simulink model "clarck"  (R2024a)
settings: Solver=FixedStepAuto  StartTime=0.0  StopTime=inf  RelTol=1e-3  EnableMultiTasking=on
libraries: stm32f4xxblockslib x1
settings Model: Creator=wsl  LastModifiedBy=wsl
settings SolverCC: AutoInsertRateTranBlk=on
settings OptimizationCC: EnhancedBackFolding=on  PassReuseOutputArgsAs=Individual arguments  ZeroExternalMemoryAtStartup=off  ZeroInternalMemoryAtStartup=off  MaxStackSize=64  OptimizeBlockOrder=speed  DifferentSizesBufferReuse=on  OptimizationCustomize=off  EfficientTunableParamExpr=on
settings DebuggingCC: ParameterTunabilityLossMsg=error
settings HardwareCC: ProdBitPerPointer=32  ProdBitPerSizeT=32  ProdBitPerPtrDiffT=32  ProdLargestAtomicInteger=Long  ProdLargestAtomicFloat=Double  ProdWordSize=32  ProdLongLongMode=on  ProdHWDeviceType=ARM Compatible->ARM Cortex-M
settings SFSimCC: MATLABDynamicMemAlloc=off
settings RTWCC: Description=Embedded Coder  SystemTargetFile=ert.tlc  HardwareBoard=STM32F4xx Based  TemplateMakefile=ert_default_tmf  Toolchain=GNU Tools for ARM Embedded Processors
settings CodeAppCC: ForceParamTrailComments=on  IgnoreCustomStorageClasses=off  OperatorAnnotations=on  SimulinkDataObjDesc=on  SFDataObjDesc=on  InsertBlockDesc=on
settings ERTTargetCC: TargetLangStandard=C99 (ISO)  CodeReplacementLibrary=ARM Cortex-M  ExtModeTransport=3  ExtModeStaticAlloc=on  ExtModeStaticAllocSize=2048  ExtModeMexFile=ext_xcp  ExtModeIntrfLevel=Level2 - Open

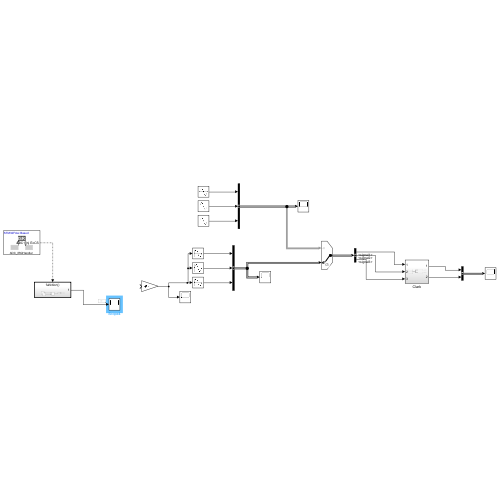
[thumbnail: Simulink's stored preview of the top-level diagram]
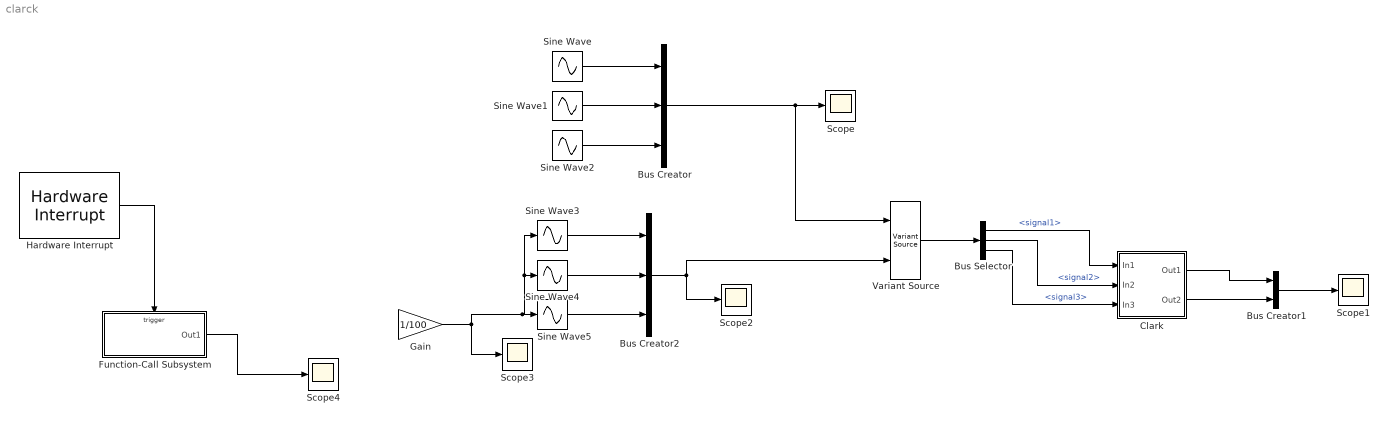
== system clarck ==
  Bus Creator : BusCreator  Inputs=3
  Bus Creator1 : BusCreator  Inputs=2
  Bus Creator2 : BusCreator  Inputs=3
  Bus Selector : BusSelector  OutputSignals=signal1,signal2,signal3
  Clark : Subsystem
  Function-Call Subsystem : Subsystem  TreatAsAtomicUnit=on
  Gain : Gain  Gain=1/100
  Hardware Interrupt : stm32f4xxblockslib/Hardware Interrupt  ISRGroup=Analog to digital converter (ADC)  ISRName=ADC_IRQHandler  ISRNumber=33  EventsList={ 'off', 'ADC1 OVR', '1'; 'off', 'ADC1 Reg EoCS', '2'; 'on', 'ADC1 Inj EoCS', '3'; 'off', 'ADC1 Watchdog', '4'; 'off', 'ADC2 OVR', '5'; 'off', 'ADC2 Reg EoCS', '6'; 'off', 'ADC2 Inj EoCS', '7'; 'off', 'ADC2 Watchdog', '8'; 'off', 'ADC3 OVR', '9'; 'off', 'ADC3 Reg EoCS', '10'; 'off', 'ADC3 Inj EoCS', '11'; 'off', 'ADC3 Watchdog', '12'; 'off', 'Custom event', '13' }  SelectedEvents={'ADC1 Inj EoCS'}  TaskPriority=30  DisablePreemption=off  ClearInterruptFlagsAtEndOfEvent=off  InterruptDefinitionFile=$(TARGET_ROOT)/registry/interrupts/STM32F4xxBased_interrupts.xml  HardwareBoard=STM32F4xx Based  EnableSimPort=off
  Scope{,1..4} (5 alike) : Scope
  Sine Wave : Sin  SineType=Sample based  Samples=1000  SampleTime=1e-4
  Sine Wave1 : Sin  SineType=Sample based  Samples=1000  SampleTime=1e-4  Offset=333
  Sine Wave2 : Sin  SineType=Sample based  Samples=1000  SampleTime=1e-4  Offset=-333
  Sine Wave3 : Sin  TimeSource=Use external signal  Frequency=2*pi  Samples=1000  SampleTime=1e-4
  Sine Wave4 : Sin  TimeSource=Use external signal  Frequency=2*pi  Phase=2/3*pi  Samples=1000  SampleTime=1e-4  Offset=333
  Sine Wave5 : Sin  TimeSource=Use external signal  Frequency=2*pi  Phase=-2/3*pi  Samples=1000  SampleTime=1e-4  Offset=-333
  Variant Source : VariantSource  VariantControlMode=sim codegen switching
  wires:
  Sine Wave/1 -> Bus Creator/1
  Bus Creator/1 -> Variant Source/1, Scope/1
  Sine Wave1/1 -> Bus Creator/2
  Sine Wave2/1 -> Bus Creator/3
  Variant Source/1 -> Bus Selector/1
  Bus Selector/1 -> Clark/1(In1)  "<signal1>"
  Bus Selector/2 -> Clark/2(In2)  "<signal2>"
  Bus Selector/3 -> Clark/3(In3)  "<signal3>"
  Clark/1(Out1) -> Bus Creator1/1
  Clark/2(Out2) -> Bus Creator1/2
  Bus Creator1/1 -> Scope1/1
  Sine Wave3/1 -> Bus Creator2/1
  Sine Wave5/1 -> Bus Creator2/3
  Sine Wave4/1 -> Bus Creator2/2
  Bus Creator2/1 -> Variant Source/2, Scope2/1
  Function-Call Subsystem/1(Out1) -> Scope4/1
  Gain/1 -> Sine Wave4/1, Sine Wave3/1, Sine Wave5/1, Scope3/1
  Hardware Interrupt/1 -> Function-Call Subsystem/Trigger

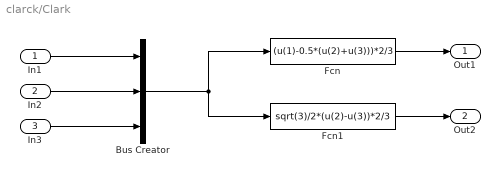
== system clarck/Clark ==
  In1 : Inport
  In2 : Inport  Port=2
  In3 : Inport  Port=3
  Bus Creator : BusCreator  Inputs=3
  Fcn : Fcn  Expr=(u(1)-0.5*(u(2)+u(3)))*2/3
  Fcn1 : Fcn  Expr=sqrt(3)/2*(u(2)-u(3))*2/3
  Out1 : Outport
  Out2 : Outport  Port=2
  wires:
  In1/1 -> Bus Creator/1
  In3/1 -> Bus Creator/3
  Fcn1/1 -> Out2/1
  In2/1 -> Bus Creator/2
  Bus Creator/1 -> Fcn1/1, Fcn/1
  Fcn/1 -> Out1/1

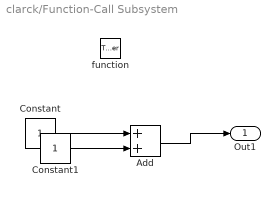
== system clarck/Function-Call Subsystem ==
  function : TriggerPort  TriggerType=function-call  VariantControl=(inherit)
  Add : Sum
  Constant : Constant
  Constant1 : Constant
  Out1 : Outport
  wires:
  Constant/1 -> Add/1
  Add/1 -> Out1/1
  Constant1/1 -> Add/2
